simulink model "four_quad_formation_270714"  (R2012b)
settings: Solver=ode5  StartTime=0.0  StopTime=inf  FixedStep=sample_time  RelTol=1e-3
InitFcn:
  | sample_time=0.005;%0.004;%0.0025;%0.02;
  | sample_time_Vicon = 0.005;
  | DeltaT = 0.02;
  | g = 9.81;
  | H0 = g%0.3165;
  | Kl = 1;
  | 
  | Q6_mass = 0.8;
  | 
  | Q6_Omega_r = 1.2; %for horizon ref
  | Q6_Zeta_r = 0.707; %for horizon ref
  | Q6_Omega_r_h = 2;%for vertical ref
  | Q6_Zeta_r_h = 0.7; %for vertical ref
  | 
  | 
  | Q6_Omega = 1.5; %for horizon control
  | Q6_Zeta = 0.507; %for horizon control
  | Q6_Omega_h= 2 %for vertical control
  | Q6_Zeta_h = 0.5; %for vertical control
  | 
  | 
  | Q6_acc_max = 5;%horizontal max acc
  | Q6_acc_max_h = 5;%horizontal max acc
  | 
  | omega_circle = 10*pi/180;
  | 
  | omega_h = 0.1;%Ascending speed
  | PI = pi;
  | Circle_R = 2;
  | 
  | 
  | MAX_Height = -2;
  | 
  | 
  | % for NN
  | n = 5;
  | r = 3;
  | n2 = 5;
  | NN_ST = 0.02;
  | 
  | GAMA_V = 6;
  | gama_V_e = 0.01;
  | 
  | GAMA_W = GAMA_V;
  | gama_W_e =0.01;
  | 
  | % deadzone
  | NN_Deadzone_Z = 0;
  | 
  | % inputs nomalizaton parameters
  | NN_Z_y_min = -3;
  | NN_Z_y_max = 0.5;
  | 
  | NN_Z_v_max = 8;
  | NN_Z_v_min = -NN_Z_v_max;
  | 
  | % alpha = 0.034;
  | alpha = 1;
  | % c_f = 0.0015;
  | c_f = 0.001;
  | c_y_tilt = 1*0.5;
libraries: X330_Control x20, simulink x8
settings Model: Creator=ttcl3  LastModifiedBy=Vicon
settings SolverCC: MaxConsecutiveMinStep=auto
settings DataIOCC: SignalLoggingSaveFormat=ModelDataLogs
settings DebuggingCC: MultiTaskRateTransMsg=warning  FcnCallInpInsideContextMsg=UseLocalSettings
settings SFSimCC: SimParseCustomCode=off
settings GRTTargetCC: CombineOutputUpdateFcns=off  GRTInterface=on

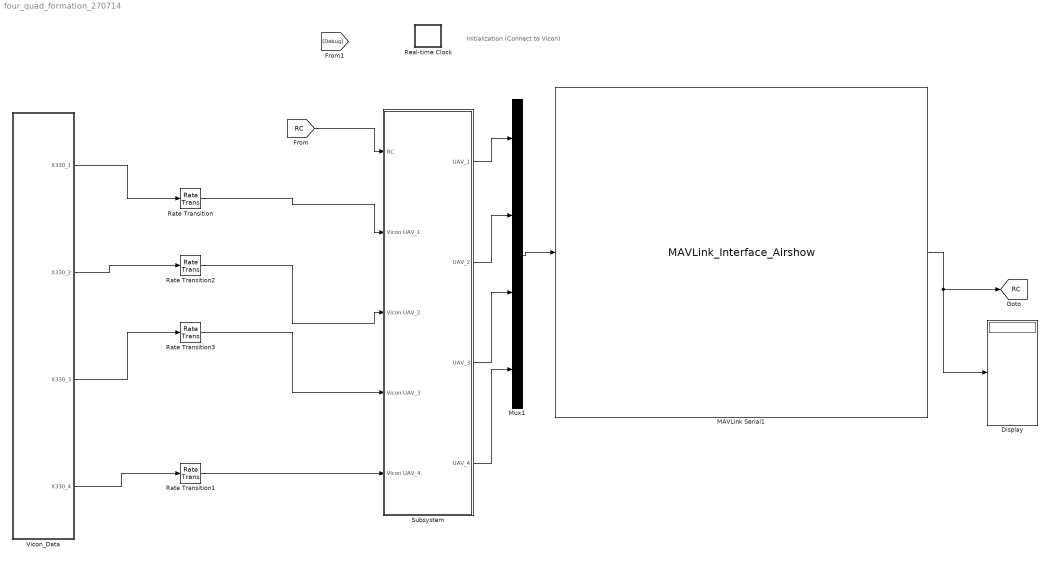
== system four_quad_formation_270714 ==
  note: Initialization
      | (Connect to Vicon)
  Display : Display
  MAVLink Serial1 : S-Function  FunctionName=MAVLink_Interface_Airshow  Parameters=COM_Port,Baud_Rate,MSG_INPUT,MSG_OUTPUT  EnableBusSupport=off  mask{COM_Port='COM6', Baud_Rate=57600, ATTITUDE_OUT=off, RC_SCALED=on, Quads_1=off, Quads_2=off, Quads_3=off, Quads_4=on, Quads_5=off, Quads_6=off}
      mask prompts: COM_Port "COM Port"; Baud_Rate "Baud Rate"; ATTITUDE_OUT "DEBUG"; RC_SCALED "RC CHANNELS SCALED"; Quads_1 "1 Quad"; Quads_2 "2 Quad"; Quads_3 "3 Quad"; Quads_4 "4 Quad"; Quads_5 "5 Quad"; Quads_6 "6 Quad"
      mask init:
      | MSG_ID_NUM_INPUT = [ uint8(221) uint8(222) uint8(223) uint8(224) uint8(225) uint8(226)];
      | MSG_ID_NAME_INPUT = [Quads_1 Quads_2 Quads_3 Quads_4 Quads_5 Quads_6];
      | 
      | MSG_ID_NUM_OUTPUT = [uint8(34) uint8(30)];
      | MSG_ID_NAME_OUTPUT = [RC_SCALED ATTITUDE_OUT ];
      | 
      | idx_input = find(MSG_ID_NAME_INPUT);
      | MSG_INPUT = MSG_ID_NUM_INPUT(idx_input);
      | 
      | idx_output = find(MSG_ID_NAME_OUTPUT);
      | MSG_OUTPUT = MSG_ID_NUM_OUTPUT(idx_output);
      mask Display:
      | % Block image
      | image(imread('10-inch Quad Heat Map.png'));
      | 
      | %Label block
      | fprintf('MAVLink Serial\n%s\n%dbps', COM_Port,  Baud_Rate)
      | 
      | 
      | %Label input ports
      | 
      | in = 1;
      | if (Quads_1 == 1)
      |     port_label('input', in, 'Quads_1');
      |     in = in + 1;
      | end
      | 
      | if (Quads_2 == 1)
      |     port_label('input', in, 'Quads_2');
      |     in = in + 1;
      | end
      | 
      | if (Quads_3 == 1)
      |     port_label('input', in, 'Quads_3');
      |     in = in + 1;
      | end
      | 
      | if (Quads_4 == 1)
      |     port_label('input', in, 'Quads_4');
      |     in = in + 1;
      | end
      | 
      | if (Quads_5 == 1)
      |     port_label('input', in, 'Quads_5');
      |     in = in + 1;
      | end
      | 
      | 
      | if (Quads_6 == 1)
      |     port_label('input', in, 'Quads_6');
      |     in = in + 1;
      | end
      | %Label output ports
      | 
      | out = 1;
      | if (RC_SCALED == 1)
      |     port_label('output', out, 'RC CMD');
      |     out = out + 1;
      | end
      | 
      | if (ATTITUDE_OUT == 1)
      |     port_label('output', out, 'DEBUG');
      |     out = out + 1;
      | end
  Mux1 : Mux
  Rate Transition{,1..3} (4 alike) : RateTransition  OutPortSampleTime=0.02
  Real-time Clock : Subsystem  mask(Real-time Clock){sample_time=0.02, tolerance=1}
      mask prompts: sample_time "Synchronize with real-time every n seconds:"; tolerance "Real-time warning tolerance (seconds):"
      mask help: Real-time Synchronization Block
      mask Help: This block synchronizes simulation time with the PC real-time clock or UNIX system clock. The first dialog entry is the period at which the clock is checked to insure real-time synchronization. The second dialog entry is the number of seconds that the simulation time must be within real-time before a warning is printed.
      mask Display: plot(0,0,100,100,[40,60,60,54,54,64,69,76,82,77,81,83,83,81,78,74,70,64,57,49,41,35,32,30,30,31,34,40,47,47,40,40],[90,90,85,85,80,79,76,87,80,70,64,57,49,41,33,28,24,22,21,23,25,31,37,46,56,65,73,78,80,85,85,90],[69,53,53],[64,50,73])
  Subsystem : Subsystem
  Vicon_Data : Subsystem
  tag scope: RC=global
  wires:
  MAVLink Serial1/1 -> [RC], Display/1
  Mux1/1 -> MAVLink Serial1/1
  Vicon_Data/1(X330_1) -> Rate Transition/1
  Vicon_Data/2(X330_2) -> Rate Transition2/1
  Vicon_Data/3(X330_3) -> Rate Transition3/1
  Rate Transition/1 -> Subsystem/2(Vicon UAV_1)
  [RC] -> Subsystem/1(RC)
  Rate Transition2/1 -> Subsystem/3(Vicon UAV_2)
  Rate Transition3/1 -> Subsystem/4(Vicon UAV_3)
  Subsystem/1(UAV_1) -> Mux1/1
  Subsystem/2(UAV_2) -> Mux1/2
  Subsystem/3(UAV_3) -> Mux1/3
  Rate Transition1/1 -> Subsystem/5(Vicon UAV_4)
  Vicon_Data/4(X330_4) -> Rate Transition1/1
  Subsystem/4(UAV_4) -> Mux1/4

== system four_quad_formation_270714/Real-time Clock ==
  Real-time Clock : S-Function  FunctionName=rtclock  Parameters=sample_time, tolerance  EnableBusSupport=off

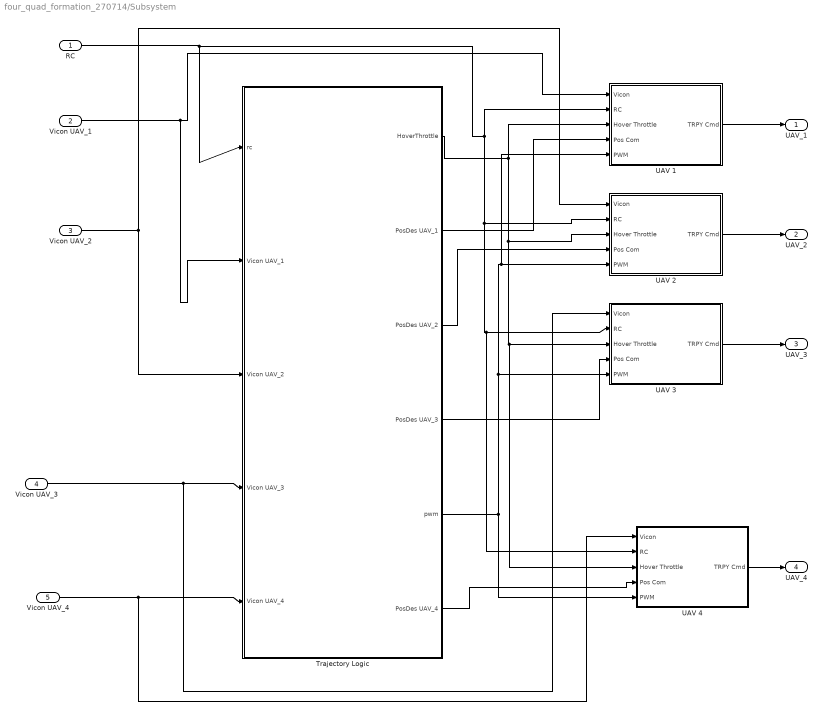
== system four_quad_formation_270714/Subsystem ==
  RC : Inport
  Vicon UAV_1 : Inport  Port=2
  Vicon UAV_2 : Inport  Port=3
  Vicon UAV_3 : Inport  Port=4
  Vicon UAV_4 : Inport  Port=5
  Trajectory Logic : Subsystem
  UAV 1 : Subsystem
  UAV 2 : Subsystem
  UAV 3 : Subsystem
  UAV 4 : Subsystem
  UAV_1 : Outport
  UAV_2 : Outport  Port=2
  UAV_3 : Outport  Port=3
  UAV_4 : Outport  Port=4
  wires:
  RC/1 -> Trajectory Logic/1(rc), UAV 1/2(RC), UAV 4/2(RC), UAV 3/2(RC), UAV 2/2(RC)
  Vicon UAV_1/1 -> UAV 1/1(Vicon), Trajectory Logic/2(Vicon UAV_1)
  UAV 1/1(TRPY Cmd) -> UAV_1/1
  Trajectory Logic/1(HoverThrottle) -> UAV 1/3(Hover Throttle), UAV 4/3(Hover Throttle), UAV 3/3(Hover Throttle), UAV 2/3(Hover Throttle)
  Trajectory Logic/2(PosDes UAV_1) -> UAV 1/4(Pos Com)
  Vicon UAV_2/1 -> Trajectory Logic/3(Vicon UAV_2), UAV 2/1(Vicon)
  Vicon UAV_3/1 -> UAV 3/1(Vicon), Trajectory Logic/4(Vicon UAV_3)
  Trajectory Logic/3(PosDes UAV_2) -> UAV 2/4(Pos Com)
  Trajectory Logic/4(PosDes UAV_3) -> UAV 3/4(Pos Com)
  UAV 2/1(TRPY Cmd) -> UAV_2/1
  UAV 3/1(TRPY Cmd) -> UAV_3/1
  Trajectory Logic/5(pwm) -> UAV 4/5(PWM), UAV 1/5(PWM), UAV 2/5(PWM), UAV 3/5(PWM)
  UAV 4/1(TRPY Cmd) -> UAV_4/1
  Vicon UAV_4/1 -> UAV 4/1(Vicon), Trajectory Logic/5(Vicon UAV_4)
  Trajectory Logic/6(PosDes UAV_4) -> UAV 4/4(Pos Com)

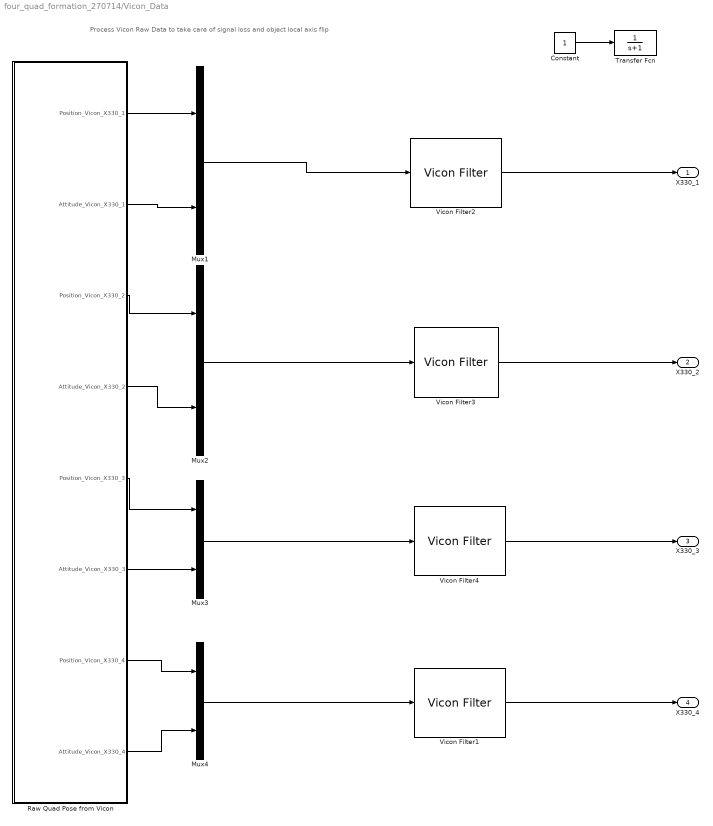
== system four_quad_formation_270714/Vicon_Data ==
  note: Process Vicon Raw Data to take care of signal loss and object local axis flip
  Constant : Constant  SampleTime=5
  Mux{1..4} (4 alike) : Mux  Inputs=2
  Raw Quad Pose from Vicon : Subsystem
  Transfer Fcn : TransferFcn  Denominator=[1 1]
  Vicon Filter{1..4} (4 alike) : X330_Control/Vicon Filter
  X330_1 : Outport
  X330_2 : Outport  Port=2
  X330_3 : Outport  Port=3
  X330_4 : Outport  Port=4
  wires:
  Vicon Filter2/1 -> X330_1/1
  Vicon Filter3/1 -> X330_2/1
  Vicon Filter4/1 -> X330_3/1
  Constant/1 -> Transfer Fcn/1
  Raw Quad Pose from Vicon/1(Position_Vicon_X330_1) -> Mux1/1
  Raw Quad Pose from Vicon/2(Attitude_Vicon_X330_1) -> Mux1/2
  Raw Quad Pose from Vicon/3(Position_Vicon_X330_2) -> Mux2/1
  Raw Quad Pose from Vicon/4(Attitude_Vicon_X330_2) -> Mux2/2
  Raw Quad Pose from Vicon/5(Position_Vicon_X330_3) -> Mux3/1
  Raw Quad Pose from Vicon/6(Attitude_Vicon_X330_3) -> Mux3/2
  Mux1/1 -> Vicon Filter2/1
  Mux2/1 -> Vicon Filter3/1
  Mux3/1 -> Vicon Filter4/1
  Vicon Filter1/1 -> X330_4/1
  Mux4/1 -> Vicon Filter1/1
  Raw Quad Pose from Vicon/7(Position_Vicon_X330_4) -> Mux4/1
  Raw Quad Pose from Vicon/8(Attitude_Vicon_X330_4) -> Mux4/2

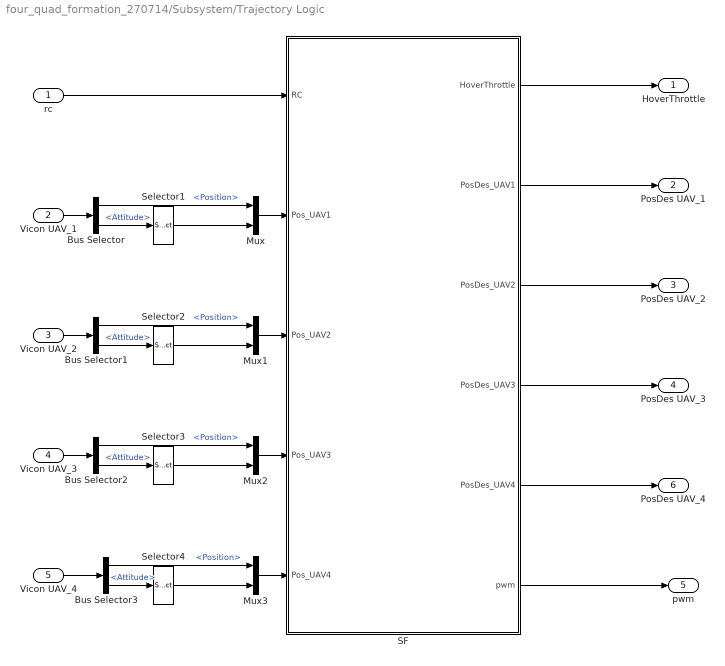
== system four_quad_formation_270714/Subsystem/Trajectory Logic ==
  rc : Inport
  Vicon UAV_1 : Inport  Port=2
  Vicon UAV_2 : Inport  Port=3
  Vicon UAV_3 : Inport  Port=4
  Vicon UAV_4 : Inport  Port=5
  " SF" : Stateflow chart  TreatAsAtomicUnit=on
  Bus Selector{,1..3} (4 alike) : BusSelector  OutputSignals=Position,Attitude
  Mux{,1..3} (4 alike) : Mux  Inputs=2
  Selector{1..4} (4 alike) : Selector  InputPortWidth=3  IndexOptions=Index vector (dialog)  Indices=[3]  OutputSizes=1
  HoverThrottle : Outport
  PosDes UAV_1 : Outport  Port=2
  PosDes UAV_2 : Outport  Port=3
  PosDes UAV_3 : Outport  Port=4
  pwm : Outport  Port=5
  PosDes UAV_4 : Outport  Port=6
  wires:
  Mux/1 -> " SF"/2(Pos_UAV1)
  Selector1/1 -> Mux/2
  Bus Selector/2 -> Selector1/1  "<Attitude>"
  Bus Selector/1 -> Mux/1  "<Position>"
  " SF"/1(HoverThrottle) -> HoverThrottle/1
  rc/1 -> " SF"/1(RC)
  " SF"/2(PosDes_UAV1) -> PosDes UAV_1/1
  Vicon UAV_1/1 -> Bus Selector/1
  Mux1/1 -> " SF"/3(Pos_UAV2)
  Selector2/1 -> Mux1/2
  Bus Selector1/2 -> Selector2/1  "<Attitude>"
  Bus Selector1/1 -> Mux1/1  "<Position>"
  Vicon UAV_2/1 -> Bus Selector1/1
  Selector3/1 -> Mux2/2
  Bus Selector2/2 -> Selector3/1  "<Attitude>"
  Bus Selector2/1 -> Mux2/1  "<Position>"
  Vicon UAV_3/1 -> Bus Selector2/1
  Mux2/1 -> " SF"/4(Pos_UAV3)
  " SF"/3(PosDes_UAV2) -> PosDes UAV_2/1
  " SF"/4(PosDes_UAV3) -> PosDes UAV_3/1
  " SF"/6(pwm) -> pwm/1
  Selector4/1 -> Mux3/2
  Bus Selector3/2 -> Selector4/1  "<Attitude>"
  Bus Selector3/1 -> Mux3/1  "<Position>"
  Vicon UAV_4/1 -> Bus Selector3/1
  Mux3/1 -> " SF"/5(Pos_UAV4)
  " SF"/5(PosDes_UAV4) -> PosDes UAV_4/1

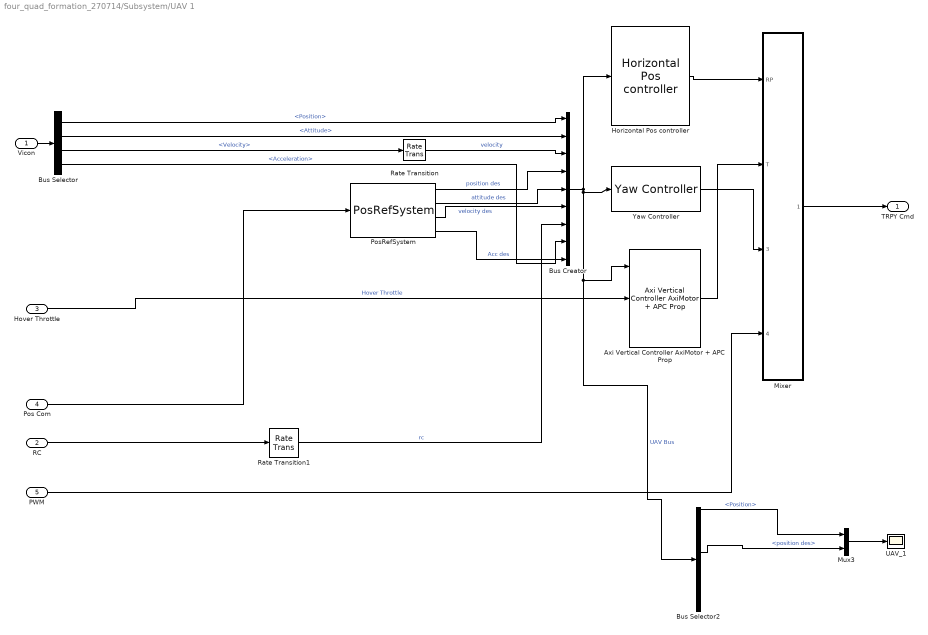
== system four_quad_formation_270714/Subsystem/UAV 1 ==
  Vicon : Inport
  RC : Inport  Port=2
  Hover Throttle : Inport  Port=3
  Pos Com : Inport  Port=4
  PWM : Inport  Port=5
  Axi Vertical Controller AxiMotor + APC Prop : X330_Control/Axi Vertical Controller AxiMotor + APC Prop  Omega_h=Q6_Omega_h  Zeta_h=Q6_Zeta_h  PID_I_h=1  mass=Q6_mass
  Bus Creator : BusCreator  Inputs=9
  Bus Selector : BusSelector  OutputSignals=Position,Attitude,Velocity,Acceleration
  Bus Selector2 : BusSelector  OutputSignals=Position,Attitude,velocity,position des,attitude des,velocity des,rc,Acc des
  Horizontal Pos controller : X330_Control/Horizontal Pos controller  Max_RP=60  Omega=Q6_Omega  PID_i=0.5  Zeta=Q6_Zeta
  Mixer : Subsystem
  Mux3 : Mux  Inputs=2
  PosRefSystem : X330_Control/PosRefSystem  Omega_r=Q6_Omega_r  Zeta_r=Q6_Zeta_r  Acc_Max=Q6_acc_max  Omega_h_r=Q6_Omega_r_h  Zeta_h_r=Q6_Zeta_r_h  Acc_h_Max=Q6_acc_max_h
      link override Saturation: LowerLimit=-3.0
  Rate Transition : RateTransition  OutPortSampleTime=0.02
  Rate Transition1 : RateTransition  OutPortSampleTime=0.02
  UAV_1 : Scope
      settings: TimeRange=10  YMin=-2.5  YMax=2
  Yaw Controller : X330_Control/Yaw Controller
  TRPY Cmd : Outport
  wires:
  Mux3/1 -> UAV_1/1
  Bus Selector2/4 -> Mux3/2  "<position des>"
  Bus Selector2/1 -> Mux3/1  "<Position>"
  RC/1 -> Rate Transition1/1
  PosRefSystem/4 -> Bus Creator/9  "Acc des"
  Vicon/1 -> Bus Selector/1
  Bus Selector/3 -> Rate Transition/1  "<Velocity>"
  Bus Selector/2 -> Bus Creator/2  "<Attitude>"
  Bus Selector/1 -> Bus Creator/1  "<Position>"
  Hover Throttle/1 -> Axi Vertical Controller AxiMotor + APC Prop/2  "Hover Throttle"
  PosRefSystem/3 -> Bus Creator/6  "velocity des"
  PosRefSystem/2 -> Bus Creator/5  "attitude des"
  PosRefSystem/1 -> Bus Creator/4  "position des"
  Bus Selector/4 -> Bus Creator/8  "<Acceleration>"
  Axi Vertical Controller AxiMotor + APC Prop/1 -> Mixer/2(T)
  Yaw Controller/1 -> Mixer/3(Yaw rate)
  Bus Creator/1 -> Yaw Controller/1, Bus Selector2/1, Axi Vertical Controller AxiMotor + APC Prop/1, Horizontal Pos controller/1  "UAV Bus"
  Rate Transition1/1 -> Bus Creator/7  "rc"
  Rate Transition/1 -> Bus Creator/3  "velocity"
  Horizontal Pos controller/1 -> Mixer/1(RP)
  Mixer/1(UAV_1) -> TRPY Cmd/1
  Pos Com/1 -> PosRefSystem/1
  PWM/1 -> Mixer/4(PWM)

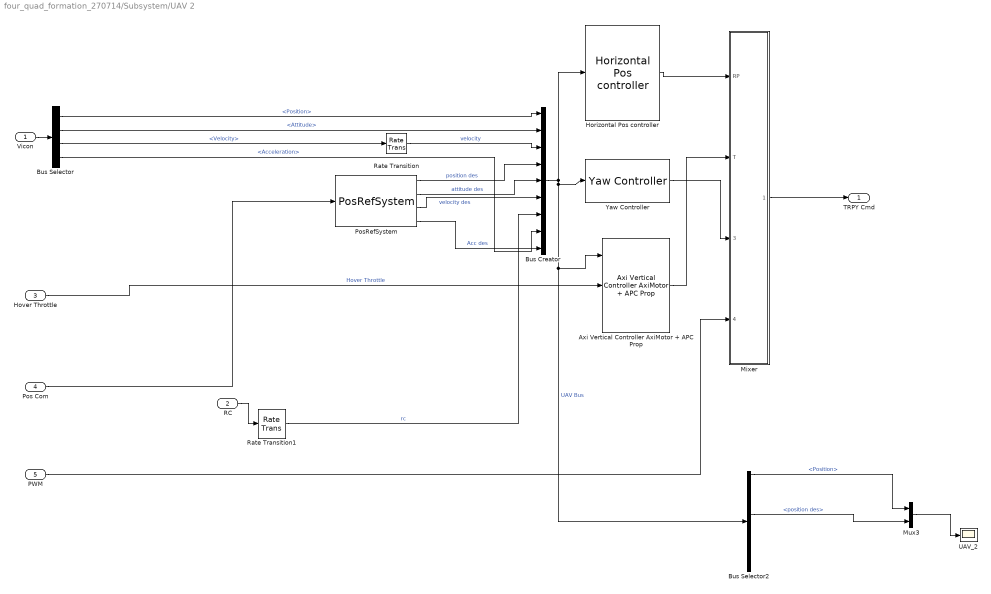
== system four_quad_formation_270714/Subsystem/UAV 2 ==
  Vicon : Inport
  RC : Inport  Port=2
  Hover Throttle : Inport  Port=3
  Pos Com : Inport  Port=4
  PWM : Inport  Port=5
  Axi Vertical Controller AxiMotor + APC Prop : X330_Control/Axi Vertical Controller AxiMotor + APC Prop  Omega_h=Q6_Omega_h  Zeta_h=Q6_Zeta_h  PID_I_h=1  mass=Q6_mass
  Bus Creator : BusCreator  Inputs=9
  Bus Selector : BusSelector  OutputSignals=Position,Attitude,Velocity,Acceleration
  Bus Selector2 : BusSelector  OutputSignals=Position,Attitude,velocity,position des,attitude des,velocity des,rc,Acc des
  Horizontal Pos controller : X330_Control/Horizontal Pos controller  Max_RP=60  Omega=Q6_Omega  PID_i=0.5  Zeta=Q6_Zeta
  Mixer : Subsystem
  Mux3 : Mux  Inputs=2
  PosRefSystem : X330_Control/PosRefSystem  Omega_r=Q6_Omega_r  Zeta_r=Q6_Zeta_r  Acc_Max=Q6_acc_max  Omega_h_r=Q6_Omega_r_h  Zeta_h_r=Q6_Zeta_r_h  Acc_h_Max=Q6_acc_max_h
      link override Saturation: LowerLimit=-3.0
  Rate Transition : RateTransition  OutPortSampleTime=0.02
  Rate Transition1 : RateTransition  OutPortSampleTime=0.02
  UAV_2 : Scope
      settings: TimeRange=10  YMin=-0.55  YMax=0.1  SaveName=ScopeData2
  Yaw Controller : X330_Control/Yaw Controller
  TRPY Cmd : Outport
  wires:
  Pos Com/1 -> PosRefSystem/1
  Mixer/1(UAV_1) -> TRPY Cmd/1
  Horizontal Pos controller/1 -> Mixer/1(RP)
  Rate Transition/1 -> Bus Creator/3  "velocity"
  Rate Transition1/1 -> Bus Creator/7  "rc"
  Yaw Controller/1 -> Mixer/3(Yaw rate)
  Axi Vertical Controller AxiMotor + APC Prop/1 -> Mixer/2(T)
  Bus Selector/4 -> Bus Creator/8  "<Acceleration>"
  PosRefSystem/1 -> Bus Creator/4  "position des"
  PosRefSystem/2 -> Bus Creator/5  "attitude des"
  PosRefSystem/3 -> Bus Creator/6  "velocity des"
  Hover Throttle/1 -> Axi Vertical Controller AxiMotor + APC Prop/2  "Hover Throttle"
  Bus Selector/1 -> Bus Creator/1  "<Position>"
  Bus Selector/2 -> Bus Creator/2  "<Attitude>"
  Bus Selector/3 -> Rate Transition/1  "<Velocity>"
  Vicon/1 -> Bus Selector/1
  PosRefSystem/4 -> Bus Creator/9  "Acc des"
  RC/1 -> Rate Transition1/1
  PWM/1 -> Mixer/4(PWM)
  Mux3/1 -> UAV_2/1
  Bus Selector2/4 -> Mux3/2  "<position des>"
  Bus Selector2/1 -> Mux3/1  "<Position>"
  Bus Creator/1 -> Horizontal Pos controller/1, Bus Selector2/1, Axi Vertical Controller AxiMotor + APC Prop/1, Yaw Controller/1  "UAV Bus"

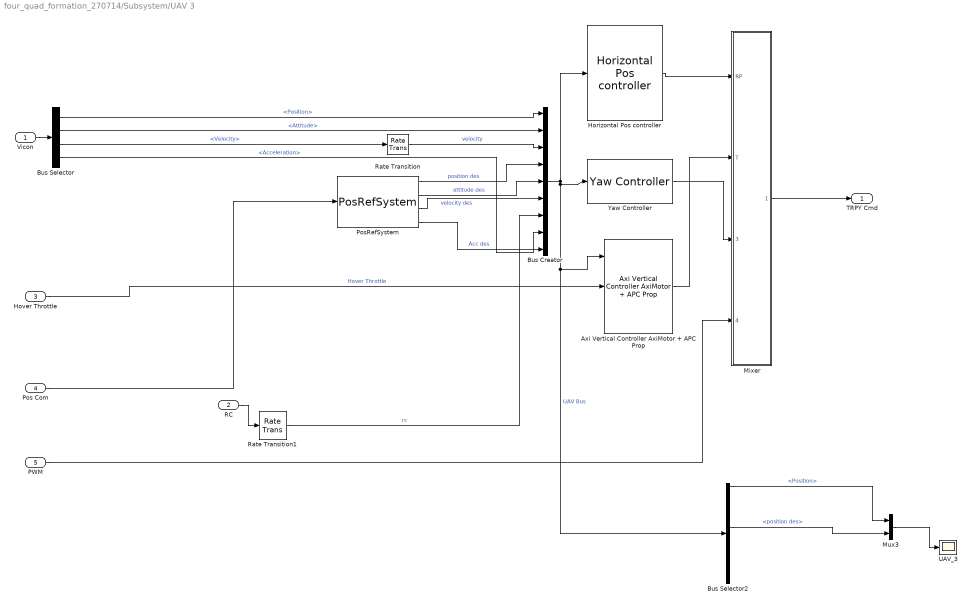
== system four_quad_formation_270714/Subsystem/UAV 3 ==
  Vicon : Inport
  RC : Inport  Port=2
  Hover Throttle : Inport  Port=3
  Pos Com : Inport  Port=4
  PWM : Inport  Port=5
  Axi Vertical Controller AxiMotor + APC Prop : X330_Control/Axi Vertical Controller AxiMotor + APC Prop  Omega_h=Q6_Omega_h  Zeta_h=Q6_Zeta_h  PID_I_h=1  mass=Q6_mass
  Bus Creator : BusCreator  Inputs=9
  Bus Selector : BusSelector  OutputSignals=Position,Attitude,Velocity,Acceleration
  Bus Selector2 : BusSelector  OutputSignals=Position,Attitude,velocity,position des,attitude des,velocity des,rc,Acc des
  Horizontal Pos controller : X330_Control/Horizontal Pos controller  Max_RP=60  Omega=Q6_Omega  PID_i=0.5  Zeta=Q6_Zeta
  Mixer : Subsystem
  Mux3 : Mux  Inputs=2
  PosRefSystem : X330_Control/PosRefSystem  Omega_r=Q6_Omega_r  Zeta_r=Q6_Zeta_r  Acc_Max=Q6_acc_max  Omega_h_r=Q6_Omega_r_h  Zeta_h_r=Q6_Zeta_r_h  Acc_h_Max=Q6_acc_max_h
      link override Saturation: LowerLimit=-3.0
  Rate Transition : RateTransition  OutPortSampleTime=0.02
  Rate Transition1 : RateTransition  OutPortSampleTime=0.02
  UAV_3 : Scope
      settings: TimeRange=10  YMin=-1.7  YMax=0
  Yaw Controller : X330_Control/Yaw Controller
  TRPY Cmd : Outport
  wires:
  RC/1 -> Rate Transition1/1
  PosRefSystem/4 -> Bus Creator/9  "Acc des"
  Vicon/1 -> Bus Selector/1
  Bus Selector/3 -> Rate Transition/1  "<Velocity>"
  Bus Selector/2 -> Bus Creator/2  "<Attitude>"
  Bus Selector/1 -> Bus Creator/1  "<Position>"
  Hover Throttle/1 -> Axi Vertical Controller AxiMotor + APC Prop/2  "Hover Throttle"
  PosRefSystem/3 -> Bus Creator/6  "velocity des"
  PosRefSystem/2 -> Bus Creator/5  "attitude des"
  PosRefSystem/1 -> Bus Creator/4  "position des"
  Bus Selector/4 -> Bus Creator/8  "<Acceleration>"
  Axi Vertical Controller AxiMotor + APC Prop/1 -> Mixer/2(T)
  Yaw Controller/1 -> Mixer/3(Yaw rate)
  Rate Transition1/1 -> Bus Creator/7  "rc"
  Rate Transition/1 -> Bus Creator/3  "velocity"
  Horizontal Pos controller/1 -> Mixer/1(RP)
  Mixer/1(UAV_1) -> TRPY Cmd/1
  Pos Com/1 -> PosRefSystem/1
  PWM/1 -> Mixer/4(PWM)
  Mux3/1 -> UAV_3/1
  Bus Selector2/4 -> Mux3/2  "<position des>"
  Bus Selector2/1 -> Mux3/1  "<Position>"
  Bus Creator/1 -> Yaw Controller/1, Bus Selector2/1, Axi Vertical Controller AxiMotor + APC Prop/1, Horizontal Pos controller/1  "UAV Bus"

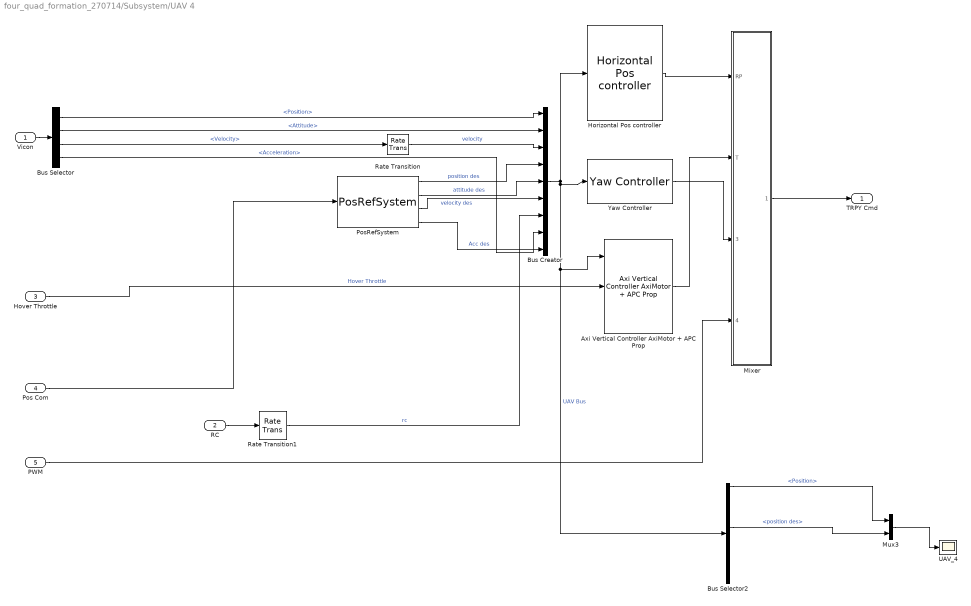
== system four_quad_formation_270714/Subsystem/UAV 4 ==
  Vicon : Inport
  RC : Inport  Port=2
  Hover Throttle : Inport  Port=3
  Pos Com : Inport  Port=4
  PWM : Inport  Port=5
  Axi Vertical Controller AxiMotor + APC Prop : X330_Control/Axi Vertical Controller AxiMotor + APC Prop  Omega_h=Q6_Omega_h  Zeta_h=Q6_Zeta_h  PID_I_h=1  mass=Q6_mass
  Bus Creator : BusCreator  Inputs=9
  Bus Selector : BusSelector  OutputSignals=Position,Attitude,Velocity,Acceleration
  Bus Selector2 : BusSelector  OutputSignals=Position,Attitude,velocity,position des,attitude des,velocity des,rc,Acc des
  Horizontal Pos controller : X330_Control/Horizontal Pos controller  Max_RP=60  Omega=Q6_Omega  PID_i=0.5  Zeta=Q6_Zeta
  Mixer : Subsystem
  Mux3 : Mux  Inputs=2
  PosRefSystem : X330_Control/PosRefSystem  Omega_r=Q6_Omega_r  Zeta_r=Q6_Zeta_r  Acc_Max=Q6_acc_max  Omega_h_r=Q6_Omega_r_h  Zeta_h_r=Q6_Zeta_r_h  Acc_h_Max=Q6_acc_max_h
      link override Saturation: LowerLimit=-3.0
  Rate Transition : RateTransition  OutPortSampleTime=0.02
  Rate Transition1 : RateTransition  OutPortSampleTime=0.02
  UAV_4 : Scope
      settings: TimeRange=10  YMin=-2.75  YMax=2.25
  Yaw Controller : X330_Control/Yaw Controller
  TRPY Cmd : Outport
  wires:
  Bus Creator/1 -> Horizontal Pos controller/1, Axi Vertical Controller AxiMotor + APC Prop/1, Bus Selector2/1, Yaw Controller/1  "UAV Bus"
  Bus Selector2/1 -> Mux3/1  "<Position>"
  Bus Selector2/4 -> Mux3/2  "<position des>"
  Mux3/1 -> UAV_4/1
  PWM/1 -> Mixer/4(PWM)
  Pos Com/1 -> PosRefSystem/1
  Mixer/1(UAV_1) -> TRPY Cmd/1
  Horizontal Pos controller/1 -> Mixer/1(RP)
  Rate Transition/1 -> Bus Creator/3  "velocity"
  Rate Transition1/1 -> Bus Creator/7  "rc"
  Yaw Controller/1 -> Mixer/3(Yaw rate)
  Axi Vertical Controller AxiMotor + APC Prop/1 -> Mixer/2(T)
  Bus Selector/4 -> Bus Creator/8  "<Acceleration>"
  PosRefSystem/1 -> Bus Creator/4  "position des"
  PosRefSystem/2 -> Bus Creator/5  "attitude des"
  PosRefSystem/3 -> Bus Creator/6  "velocity des"
  Hover Throttle/1 -> Axi Vertical Controller AxiMotor + APC Prop/2  "Hover Throttle"
  Bus Selector/1 -> Bus Creator/1  "<Position>"
  Bus Selector/2 -> Bus Creator/2  "<Attitude>"
  Bus Selector/3 -> Rate Transition/1  "<Velocity>"
  Vicon/1 -> Bus Selector/1
  PosRefSystem/4 -> Bus Creator/9  "Acc des"
  RC/1 -> Rate Transition1/1

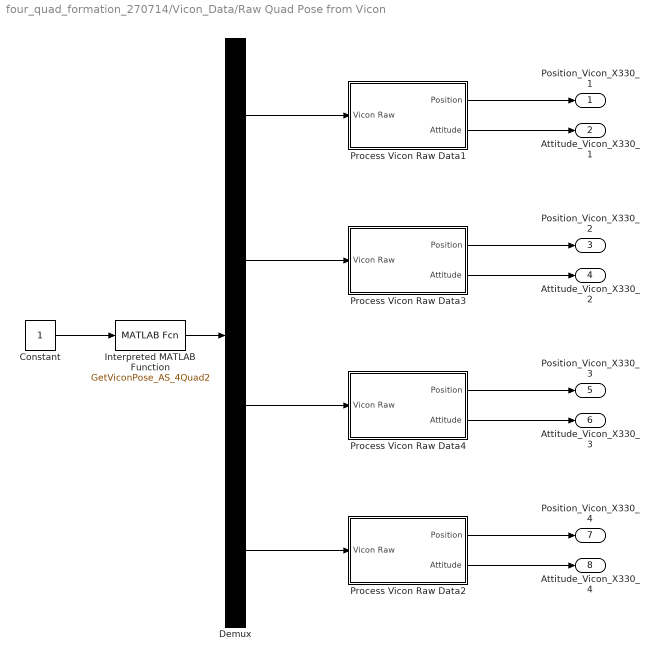
== system four_quad_formation_270714/Vicon_Data/Raw Quad Pose from Vicon ==
  Constant : Constant  SampleTime=sample_time
  Demux : Demux
  Interpreted MATLAB Function : MATLABFcn  MATLABFcn=GetViconPose_AS_4Quad2
  Process Vicon Raw Data1 : Subsystem
  Process Vicon Raw Data2 : Subsystem
  Process Vicon Raw Data3 : Subsystem
  Process Vicon Raw Data4 : Subsystem
  Position_Vicon_X330_1 : Outport
  Attitude_Vicon_X330_1 : Outport  Port=2
  Position_Vicon_X330_2 : Outport  Port=3
  Attitude_Vicon_X330_2 : Outport  Port=4
  Position_Vicon_X330_3 : Outport  Port=5
  Attitude_Vicon_X330_3 : Outport  Port=6
  Position_Vicon_X330_4 : Outport  Port=7
  Attitude_Vicon_X330_4 : Outport  Port=8
  wires:
  Interpreted MATLAB Function/1 -> Demux/1
  Constant/1 -> Interpreted MATLAB Function/1
  Process Vicon Raw Data1/2(Attitude) -> Attitude_Vicon_X330_1/1
  Process Vicon Raw Data1/1(Position) -> Position_Vicon_X330_1/1
  Process Vicon Raw Data3/2(Attitude) -> Attitude_Vicon_X330_2/1
  Process Vicon Raw Data3/1(Position) -> Position_Vicon_X330_2/1
  Process Vicon Raw Data4/2(Attitude) -> Attitude_Vicon_X330_3/1
  Process Vicon Raw Data4/1(Position) -> Position_Vicon_X330_3/1
  Demux/1 -> Process Vicon Raw Data1/1(Vicon Raw)
  Demux/2 -> Process Vicon Raw Data3/1(Vicon Raw)
  Demux/3 -> Process Vicon Raw Data4/1(Vicon Raw)
  Process Vicon Raw Data2/2(Attitude) -> Attitude_Vicon_X330_4/1
  Process Vicon Raw Data2/1(Position) -> Position_Vicon_X330_4/1
  Demux/4 -> Process Vicon Raw Data2/1(Vicon Raw)

== system four_quad_formation_270714/Subsystem/UAV 1/Mixer ==
  RP : Inport
  T : Inport  Port=2
  Yaw rate : Inport  Port=3
  PWM : Inport  Port=4
  Gain : Gain  Gain=180/pi
  Mode : Constant  SampleTime=0.02
  Mux1 : Mux  Inputs=5
  "[-1, 1]" : Fcn  Expr=u(1)*2-1
  UAV_1 : Outport
  wires:
  "[-1, 1]"/1 -> Mux1/1
  Gain/1 -> Mux1/2
  Mode/1 -> Mux1/4
  Yaw rate/1 -> Mux1/3
  RP/1 -> Gain/1
  T/1 -> "[-1, 1]"/1
  Mux1/1 -> UAV_1/1
  PWM/1 -> Mux1/5

== system four_quad_formation_270714/Subsystem/UAV 2/Mixer ==
  RP : Inport
  T : Inport  Port=2
  Yaw rate : Inport  Port=3
  PWM : Inport  Port=4
  Gain : Gain  Gain=180/pi
  Mode : Constant  SampleTime=0.02
  Mux1 : Mux  Inputs=5
  "[-1, 1]" : Fcn  Expr=u(1)*2-1
  UAV_1 : Outport
  wires:
  PWM/1 -> Mux1/5
  Mux1/1 -> UAV_1/1
  T/1 -> "[-1, 1]"/1
  RP/1 -> Gain/1
  Yaw rate/1 -> Mux1/3
  Mode/1 -> Mux1/4
  Gain/1 -> Mux1/2
  "[-1, 1]"/1 -> Mux1/1

== system four_quad_formation_270714/Subsystem/UAV 3/Mixer ==
  RP : Inport
  T : Inport  Port=2
  Yaw rate : Inport  Port=3
  PWM : Inport  Port=4
  Gain : Gain  Gain=180/pi
  Mode : Constant  SampleTime=0.02
  Mux1 : Mux  Inputs=5
  "[-1, 1]" : Fcn  Expr=u(1)*2-1
  UAV_1 : Outport
  wires:
  "[-1, 1]"/1 -> Mux1/1
  Gain/1 -> Mux1/2
  Mode/1 -> Mux1/4
  Yaw rate/1 -> Mux1/3
  RP/1 -> Gain/1
  T/1 -> "[-1, 1]"/1
  Mux1/1 -> UAV_1/1
  PWM/1 -> Mux1/5

== system four_quad_formation_270714/Subsystem/UAV 4/Mixer ==
  RP : Inport
  T : Inport  Port=2
  Yaw rate : Inport  Port=3
  PWM : Inport  Port=4
  Gain : Gain  Gain=180/pi
  Mode : Constant  SampleTime=0.02
  Mux1 : Mux  Inputs=5
  "[-1, 1]" : Fcn  Expr=u(1)*2-1
  UAV_1 : Outport
  wires:
  PWM/1 -> Mux1/5
  Mux1/1 -> UAV_1/1
  T/1 -> "[-1, 1]"/1
  RP/1 -> Gain/1
  Yaw rate/1 -> Mux1/3
  Mode/1 -> Mux1/4
  Gain/1 -> Mux1/2
  "[-1, 1]"/1 -> Mux1/1

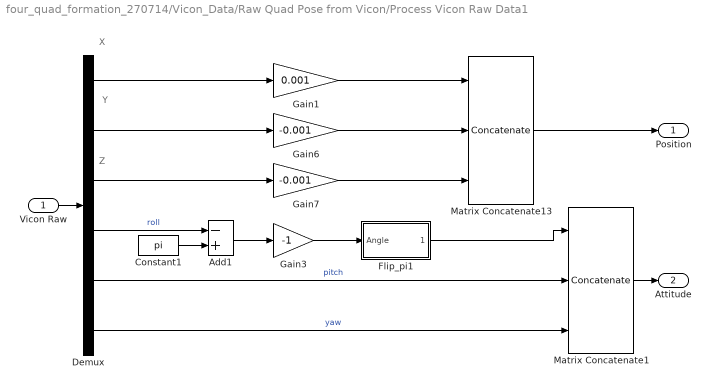
== system four_quad_formation_270714/Vicon_Data/Raw Quad Pose from Vicon/Process Vicon Raw Data1 ==
  note: X
  note: Y
  note: Z
  Vicon Raw : Inport
  Add1 : Sum  Inputs=-+
  Constant1 : Constant  Value=pi  OutDataTypeStr=double
  Demux : Demux  Outputs=6
  Flip_pi1 : Subsystem  mask(Flip -pi to pi){}
      mask help: Flips the inputs into the range -pi to pi
      mask Help: Flips the inputs into the range -pi to pi
      mask Display: disp('Flip_pi')
  Gain1 : Gain  Gain=0.001
  Gain3 : Gain  Gain=-1
  Gain6 : Gain  Gain=-0.001
  Gain7 : Gain  Gain=-0.001
  Matrix Concatenate1 : Concatenate  NumInputs=3  Mode=Multidimensional array
  Matrix Concatenate13 : Concatenate  NumInputs=3  Mode=Multidimensional array
  Position : Outport
  Attitude : Outport  Port=2
  wires:
  Constant1/1 -> Add1/2
  Demux/6 -> Matrix Concatenate1/3  "yaw"
  Gain1/1 -> Matrix Concatenate13/1
  Demux/1 -> Gain1/1
  Demux/2 -> Gain6/1
  Demux/3 -> Gain7/1
  Demux/4 -> Add1/1  "roll"
  Gain6/1 -> Matrix Concatenate13/2
  Gain7/1 -> Matrix Concatenate13/3
  Add1/1 -> Gain3/1
  Gain3/1 -> Flip_pi1/1(Angle)
  Demux/5 -> Matrix Concatenate1/2  "pitch"
  Flip_pi1/1(Angle_Flip) -> Matrix Concatenate1/1
  Matrix Concatenate13/1 -> Position/1
  Vicon Raw/1 -> Demux/1
  Matrix Concatenate1/1 -> Attitude/1

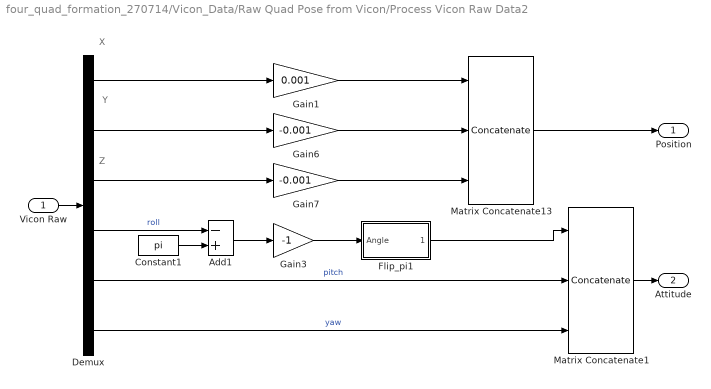
== system four_quad_formation_270714/Vicon_Data/Raw Quad Pose from Vicon/Process Vicon Raw Data2 ==
  note: Z
  note: Y
  note: X
  Vicon Raw : Inport
  Add1 : Sum  Inputs=-+
  Constant1 : Constant  Value=pi  OutDataTypeStr=double
  Demux : Demux  Outputs=6
  Flip_pi1 : Subsystem  mask(Flip -pi to pi){}
      mask help: Flips the inputs into the range -pi to pi
      mask Help: Flips the inputs into the range -pi to pi
      mask Display: disp('Flip_pi')
  Gain1 : Gain  Gain=0.001
  Gain3 : Gain  Gain=-1
  Gain6 : Gain  Gain=-0.001
  Gain7 : Gain  Gain=-0.001
  Matrix Concatenate1 : Concatenate  NumInputs=3  Mode=Multidimensional array
  Matrix Concatenate13 : Concatenate  NumInputs=3  Mode=Multidimensional array
  Position : Outport
  Attitude : Outport  Port=2
  wires:
  Matrix Concatenate1/1 -> Attitude/1
  Vicon Raw/1 -> Demux/1
  Matrix Concatenate13/1 -> Position/1
  Flip_pi1/1(Angle_Flip) -> Matrix Concatenate1/1
  Demux/5 -> Matrix Concatenate1/2  "pitch"
  Gain3/1 -> Flip_pi1/1(Angle)
  Add1/1 -> Gain3/1
  Gain7/1 -> Matrix Concatenate13/3
  Gain6/1 -> Matrix Concatenate13/2
  Demux/4 -> Add1/1  "roll"
  Demux/3 -> Gain7/1
  Demux/2 -> Gain6/1
  Demux/1 -> Gain1/1
  Gain1/1 -> Matrix Concatenate13/1
  Demux/6 -> Matrix Concatenate1/3  "yaw"
  Constant1/1 -> Add1/2

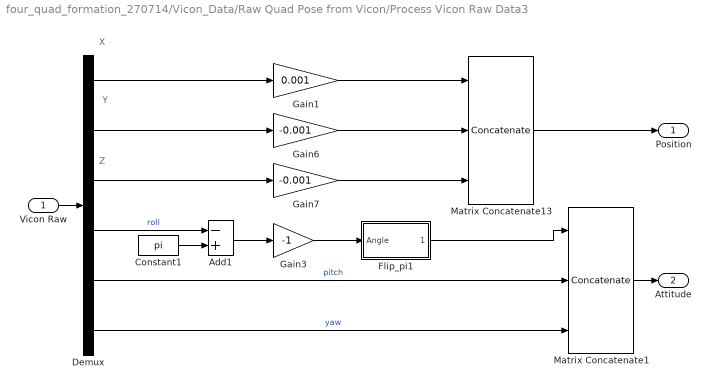
== system four_quad_formation_270714/Vicon_Data/Raw Quad Pose from Vicon/Process Vicon Raw Data3 ==
  note: Z
  note: Y
  note: X
  Vicon Raw : Inport
  Add1 : Sum  Inputs=-+
  Constant1 : Constant  Value=pi  OutDataTypeStr=double
  Demux : Demux  Outputs=6
  Flip_pi1 : Subsystem  mask(Flip -pi to pi){}
      mask help: Flips the inputs into the range -pi to pi
      mask Help: Flips the inputs into the range -pi to pi
      mask Display: disp('Flip_pi')
  Gain1 : Gain  Gain=0.001
  Gain3 : Gain  Gain=-1
  Gain6 : Gain  Gain=-0.001
  Gain7 : Gain  Gain=-0.001
  Matrix Concatenate1 : Concatenate  NumInputs=3  Mode=Multidimensional array
  Matrix Concatenate13 : Concatenate  NumInputs=3  Mode=Multidimensional array
  Position : Outport
  Attitude : Outport  Port=2
  wires:
  Matrix Concatenate1/1 -> Attitude/1
  Vicon Raw/1 -> Demux/1
  Matrix Concatenate13/1 -> Position/1
  Flip_pi1/1(Angle_Flip) -> Matrix Concatenate1/1
  Demux/5 -> Matrix Concatenate1/2  "pitch"
  Gain3/1 -> Flip_pi1/1(Angle)
  Add1/1 -> Gain3/1
  Gain7/1 -> Matrix Concatenate13/3
  Gain6/1 -> Matrix Concatenate13/2
  Demux/4 -> Add1/1  "roll"
  Demux/3 -> Gain7/1
  Demux/2 -> Gain6/1
  Demux/1 -> Gain1/1
  Gain1/1 -> Matrix Concatenate13/1
  Demux/6 -> Matrix Concatenate1/3  "yaw"
  Constant1/1 -> Add1/2

== system four_quad_formation_270714/Vicon_Data/Raw Quad Pose from Vicon/Process Vicon Raw Data4 ==
  note: X
  note: Y
  note: Z
  Vicon Raw : Inport
  Add1 : Sum  Inputs=-+
  Constant1 : Constant  Value=pi  OutDataTypeStr=double
  Demux : Demux  Outputs=6
  Flip_pi1 : Subsystem  mask(Flip -pi to pi){}
      mask help: Flips the inputs into the range -pi to pi
      mask Help: Flips the inputs into the range -pi to pi
      mask Display: disp('Flip_pi')
  Gain1 : Gain  Gain=0.001
  Gain3 : Gain  Gain=-1
  Gain6 : Gain  Gain=-0.001
  Gain7 : Gain  Gain=-0.001
  Matrix Concatenate1 : Concatenate  NumInputs=3  Mode=Multidimensional array
  Matrix Concatenate13 : Concatenate  NumInputs=3  Mode=Multidimensional array
  Position : Outport
  Attitude : Outport  Port=2
  wires:
  Constant1/1 -> Add1/2
  Demux/6 -> Matrix Concatenate1/3  "yaw"
  Gain1/1 -> Matrix Concatenate13/1
  Demux/1 -> Gain1/1
  Demux/2 -> Gain6/1
  Demux/3 -> Gain7/1
  Demux/4 -> Add1/1  "roll"
  Gain6/1 -> Matrix Concatenate13/2
  Gain7/1 -> Matrix Concatenate13/3
  Add1/1 -> Gain3/1
  Gain3/1 -> Flip_pi1/1(Angle)
  Demux/5 -> Matrix Concatenate1/2  "pitch"
  Flip_pi1/1(Angle_Flip) -> Matrix Concatenate1/1
  Matrix Concatenate13/1 -> Position/1
  Vicon Raw/1 -> Demux/1
  Matrix Concatenate1/1 -> Attitude/1

== system four_quad_formation_270714/Vicon_Data/Raw Quad Pose from Vicon/Process Vicon Raw Data1/Flip_pi1 ==
  Angle : Inport
  Add : Sum  Inputs=-+
  Compare To Constant1 : simulink/Logic and Bit Operations/Compare To Constant  relop=>  const=pi  OutDataTypeStr=uint8  ZeroCross=off
  Constant : Constant  Value=2*pi
  Data Type Duplicate : DataTypeDuplicate
  Flip_0_to_2pi : Subsystem  mask(Flip zero to 2pi){}
      mask help: Flips the inputs into the range zero to +2pi
      mask Help: Flips the inputs into the range zero to +2pi
      mask Display: disp('Flip_0_2pi')
  Switch : Switch  Criteria=u2 ~= 0
  Angle_Flip : Outport
  wires:
  Switch/1 -> Data Type Duplicate/1, Angle_Flip/1
  Add/1 -> Switch/1
  Constant/1 -> Add/1
  Compare To Constant1/1 -> Switch/2
  Flip_0_to_2pi/1(Angle_Flip) -> Add/2, Compare To Constant1/1, Switch/3
  Angle/1 -> Data Type Duplicate/2, Flip_0_to_2pi/1(Angle)

== system four_quad_formation_270714/Vicon_Data/Raw Quad Pose from Vicon/Process Vicon Raw Data2/Flip_pi1 ==
  Angle : Inport
  Add : Sum  Inputs=-+
  Compare To Constant1 : simulink/Logic and Bit Operations/Compare To Constant  relop=>  const=pi  OutDataTypeStr=uint8  ZeroCross=off
  Constant : Constant  Value=2*pi
  Data Type Duplicate : DataTypeDuplicate
  Flip_0_to_2pi : Subsystem  mask(Flip zero to 2pi){}
      mask help: Flips the inputs into the range zero to +2pi
      mask Help: Flips the inputs into the range zero to +2pi
      mask Display: disp('Flip_0_2pi')
  Switch : Switch  Criteria=u2 ~= 0
  Angle_Flip : Outport
  wires:
  Angle/1 -> Flip_0_to_2pi/1(Angle), Data Type Duplicate/2
  Flip_0_to_2pi/1(Angle_Flip) -> Switch/3, Compare To Constant1/1, Add/2
  Compare To Constant1/1 -> Switch/2
  Constant/1 -> Add/1
  Add/1 -> Switch/1
  Switch/1 -> Angle_Flip/1, Data Type Duplicate/1

== system four_quad_formation_270714/Vicon_Data/Raw Quad Pose from Vicon/Process Vicon Raw Data3/Flip_pi1 ==
  Angle : Inport
  Add : Sum  Inputs=-+
  Compare To Constant1 : simulink/Logic and Bit Operations/Compare To Constant  relop=>  const=pi  OutDataTypeStr=uint8  ZeroCross=off
  Constant : Constant  Value=2*pi
  Data Type Duplicate : DataTypeDuplicate
  Flip_0_to_2pi : Subsystem  mask(Flip zero to 2pi){}
      mask help: Flips the inputs into the range zero to +2pi
      mask Help: Flips the inputs into the range zero to +2pi
      mask Display: disp('Flip_0_2pi')
  Switch : Switch  Criteria=u2 ~= 0
  Angle_Flip : Outport
  wires:
  Angle/1 -> Flip_0_to_2pi/1(Angle), Data Type Duplicate/2
  Flip_0_to_2pi/1(Angle_Flip) -> Switch/3, Compare To Constant1/1, Add/2
  Compare To Constant1/1 -> Switch/2
  Constant/1 -> Add/1
  Add/1 -> Switch/1
  Switch/1 -> Angle_Flip/1, Data Type Duplicate/1

== system four_quad_formation_270714/Vicon_Data/Raw Quad Pose from Vicon/Process Vicon Raw Data4/Flip_pi1 ==
  Angle : Inport
  Add : Sum  Inputs=-+
  Compare To Constant1 : simulink/Logic and Bit Operations/Compare To Constant  relop=>  const=pi  OutDataTypeStr=uint8  ZeroCross=off
  Constant : Constant  Value=2*pi
  Data Type Duplicate : DataTypeDuplicate
  Flip_0_to_2pi : Subsystem  mask(Flip zero to 2pi){}
      mask help: Flips the inputs into the range zero to +2pi
      mask Help: Flips the inputs into the range zero to +2pi
      mask Display: disp('Flip_0_2pi')
  Switch : Switch  Criteria=u2 ~= 0
  Angle_Flip : Outport
  wires:
  Switch/1 -> Data Type Duplicate/1, Angle_Flip/1
  Add/1 -> Switch/1
  Constant/1 -> Add/1
  Compare To Constant1/1 -> Switch/2
  Flip_0_to_2pi/1(Angle_Flip) -> Add/2, Compare To Constant1/1, Switch/3
  Angle/1 -> Data Type Duplicate/2, Flip_0_to_2pi/1(Angle)

== system four_quad_formation_270714/Vicon_Data/Raw Quad Pose from Vicon/Process Vicon Raw Data1/Flip_pi1/Flip_0_to_2pi ==
  Angle : Inport
  Add : Sum
  Compare To Constant1 : simulink/Logic and Bit Operations/Compare To Constant  relop=<  const=0  OutDataTypeStr=uint8  ZeroCross=off
  Constant : Constant  Value=2*pi
  Data Type Duplicate : DataTypeDuplicate
  Flip_2pi : Subsystem  mask(Flip -2pi to 2pi){}
      mask help: Flips the inputs into the range -2pi to +2pi
      mask Help: Flips the inputs into the range -2pi to +2pi
      mask Display: disp('Flip_2pi')
  Switch : Switch  Criteria=u2 ~= 0
  Angle_Flip : Outport
  wires:
  Switch/1 -> Data Type Duplicate/1, Angle_Flip/1
  Angle/1 -> Data Type Duplicate/2, Flip_2pi/1(Angle)
  Add/1 -> Switch/1
  Constant/1 -> Add/1
  Compare To Constant1/1 -> Switch/2
  Flip_2pi/1(Angle_Flip) -> Switch/3, Add/2, Compare To Constant1/1

== system four_quad_formation_270714/Vicon_Data/Raw Quad Pose from Vicon/Process Vicon Raw Data2/Flip_pi1/Flip_0_to_2pi ==
  Angle : Inport
  Add : Sum
  Compare To Constant1 : simulink/Logic and Bit Operations/Compare To Constant  relop=<  const=0  OutDataTypeStr=uint8  ZeroCross=off
  Constant : Constant  Value=2*pi
  Data Type Duplicate : DataTypeDuplicate
  Flip_2pi : Subsystem  mask(Flip -2pi to 2pi){}
      mask help: Flips the inputs into the range -2pi to +2pi
      mask Help: Flips the inputs into the range -2pi to +2pi
      mask Display: disp('Flip_2pi')
  Switch : Switch  Criteria=u2 ~= 0
  Angle_Flip : Outport
  wires:
  Flip_2pi/1(Angle_Flip) -> Compare To Constant1/1, Add/2, Switch/3
  Compare To Constant1/1 -> Switch/2
  Constant/1 -> Add/1
  Add/1 -> Switch/1
  Angle/1 -> Flip_2pi/1(Angle), Data Type Duplicate/2
  Switch/1 -> Angle_Flip/1, Data Type Duplicate/1

== system four_quad_formation_270714/Vicon_Data/Raw Quad Pose from Vicon/Process Vicon Raw Data3/Flip_pi1/Flip_0_to_2pi ==
  Angle : Inport
  Add : Sum
  Compare To Constant1 : simulink/Logic and Bit Operations/Compare To Constant  relop=<  const=0  OutDataTypeStr=uint8  ZeroCross=off
  Constant : Constant  Value=2*pi
  Data Type Duplicate : DataTypeDuplicate
  Flip_2pi : Subsystem  mask(Flip -2pi to 2pi){}
      mask help: Flips the inputs into the range -2pi to +2pi
      mask Help: Flips the inputs into the range -2pi to +2pi
      mask Display: disp('Flip_2pi')
  Switch : Switch  Criteria=u2 ~= 0
  Angle_Flip : Outport
  wires:
  Flip_2pi/1(Angle_Flip) -> Compare To Constant1/1, Add/2, Switch/3
  Compare To Constant1/1 -> Switch/2
  Constant/1 -> Add/1
  Add/1 -> Switch/1
  Angle/1 -> Flip_2pi/1(Angle), Data Type Duplicate/2
  Switch/1 -> Angle_Flip/1, Data Type Duplicate/1

== system four_quad_formation_270714/Vicon_Data/Raw Quad Pose from Vicon/Process Vicon Raw Data4/Flip_pi1/Flip_0_to_2pi ==
  Angle : Inport
  Add : Sum
  Compare To Constant1 : simulink/Logic and Bit Operations/Compare To Constant  relop=<  const=0  OutDataTypeStr=uint8  ZeroCross=off
  Constant : Constant  Value=2*pi
  Data Type Duplicate : DataTypeDuplicate
  Flip_2pi : Subsystem  mask(Flip -2pi to 2pi){}
      mask help: Flips the inputs into the range -2pi to +2pi
      mask Help: Flips the inputs into the range -2pi to +2pi
      mask Display: disp('Flip_2pi')
  Switch : Switch  Criteria=u2 ~= 0
  Angle_Flip : Outport
  wires:
  Switch/1 -> Data Type Duplicate/1, Angle_Flip/1
  Angle/1 -> Data Type Duplicate/2, Flip_2pi/1(Angle)
  Add/1 -> Switch/1
  Constant/1 -> Add/1
  Compare To Constant1/1 -> Switch/2
  Flip_2pi/1(Angle_Flip) -> Switch/3, Add/2, Compare To Constant1/1

== system four_quad_formation_270714/Vicon_Data/Raw Quad Pose from Vicon/Process Vicon Raw Data1/Flip_pi1/Flip_0_to_2pi/Flip_2pi ==
  Angle : Inport
  Bias : Bias  Bias=-2*pi
  Constant : Constant  Value=2*pi
  Data Type Duplicate : DataTypeDuplicate
  Modulo : Math  Operator=mod  SaturateOnIntegerOverflow=on
  Sign1 : Signum
  Switch : Switch
  Angle_Flip : Outport
  wires:
  Switch/1 -> Data Type Duplicate/2, Angle_Flip/1
  Bias/1 -> Switch/3
  Sign1/1 -> Switch/2
  Modulo/1 -> Switch/1, Bias/1
  Constant/1 -> Modulo/2
  Angle/1 -> Data Type Duplicate/1, Sign1/1, Modulo/1

== system four_quad_formation_270714/Vicon_Data/Raw Quad Pose from Vicon/Process Vicon Raw Data2/Flip_pi1/Flip_0_to_2pi/Flip_2pi ==
  Angle : Inport
  Bias : Bias  Bias=-2*pi
  Constant : Constant  Value=2*pi
  Data Type Duplicate : DataTypeDuplicate
  Modulo : Math  Operator=mod  SaturateOnIntegerOverflow=on
  Sign1 : Signum
  Switch : Switch
  Angle_Flip : Outport
  wires:
  Angle/1 -> Modulo/1, Sign1/1, Data Type Duplicate/1
  Constant/1 -> Modulo/2
  Modulo/1 -> Bias/1, Switch/1
  Sign1/1 -> Switch/2
  Bias/1 -> Switch/3
  Switch/1 -> Angle_Flip/1, Data Type Duplicate/2

== system four_quad_formation_270714/Vicon_Data/Raw Quad Pose from Vicon/Process Vicon Raw Data3/Flip_pi1/Flip_0_to_2pi/Flip_2pi ==
  Angle : Inport
  Bias : Bias  Bias=-2*pi
  Constant : Constant  Value=2*pi
  Data Type Duplicate : DataTypeDuplicate
  Modulo : Math  Operator=mod  SaturateOnIntegerOverflow=on
  Sign1 : Signum
  Switch : Switch
  Angle_Flip : Outport
  wires:
  Angle/1 -> Modulo/1, Sign1/1, Data Type Duplicate/1
  Constant/1 -> Modulo/2
  Modulo/1 -> Bias/1, Switch/1
  Sign1/1 -> Switch/2
  Bias/1 -> Switch/3
  Switch/1 -> Angle_Flip/1, Data Type Duplicate/2

== system four_quad_formation_270714/Vicon_Data/Raw Quad Pose from Vicon/Process Vicon Raw Data4/Flip_pi1/Flip_0_to_2pi/Flip_2pi ==
  Angle : Inport
  Bias : Bias  Bias=-2*pi
  Constant : Constant  Value=2*pi
  Data Type Duplicate : DataTypeDuplicate
  Modulo : Math  Operator=mod  SaturateOnIntegerOverflow=on
  Sign1 : Signum
  Switch : Switch
  Angle_Flip : Outport
  wires:
  Switch/1 -> Data Type Duplicate/2, Angle_Flip/1
  Bias/1 -> Switch/3
  Sign1/1 -> Switch/2
  Modulo/1 -> Switch/1, Bias/1
  Constant/1 -> Modulo/2
  Angle/1 -> Data Type Duplicate/1, Sign1/1, Modulo/1

== stateflow chart four_quad_formation_270714/Subsystem/Trajectory Logic/ SF ==
  state Airborne
    state Stage6
      state Red_UAV1 [parallel]
        du:PosDes_UAV1[0] = -1.457;
        PosDes_UAV1[1] = 1.457 ;
        PosDes_UAV1[2] = -1.2;
        settings: executionOrder=1
      state Green_UAV2 [parallel]
        du:PosDes_UAV2[0] = 1.457 ;
        PosDes_UAV2[1] = 1.457;
        PosDes_UAV2[2] = -1.2;
        settings: executionOrder=2
      state PWM1 [parallel]
        du:    Increm = Increm + DeltaT
        settings: executionOrder=3
      state PWM [parallel]
        du:    pwm=  1800;
        settings: executionOrder=4
      state Blue_UAV3 [parallel]
        du:PosDes_UAV3[0] = -1.457  ;
        PosDes_UAV3[1] = -1.457;
        PosDes_UAV3[2] = -1.2;
        settings: executionOrder=5
      state Purple_UAV4 [parallel]
        du:PosDes_UAV4[0] = 1.457 ;
        PosDes_UAV4[1] = -1.457;
        PosDes_UAV4[2] = -1.2;
        settings: executionOrder=6
    state TakeOff
      du:		HoverThrottle = (H0 - HoverThrottle)*2*DeltaT + HoverThrottle ;
      PosDes_UAV1[2] = (-1.2 - PosDes_UAV1[2])*1*DeltaT + PosDes_UAV1[2] ;
      PosDes_UAV2[2] = (-1.2 - PosDes_UAV2[2])*1*DeltaT + PosDes_UAV2[2] ;
      PosDes_UAV3[2] = (-1.2 - PosDes_UAV3[2])*1*DeltaT + PosDes_UAV3[2] ;
      PosDes_UAV4[2] = (-1.2 - PosDes_UAV4[2])*1*DeltaT + PosDes_UAV4[2] ;
    state Stage1
      state Red_UAV1 [parallel]
        du:PosDes_UAV1[0] = (2- PosDes_UAV1[0])*0.75*DeltaT + PosDes_UAV1[0] ;
        PosDes_UAV1[1] = (2- PosDes_UAV1[1])*0.75*DeltaT + PosDes_UAV1[1] ;
        PosDes_UAV1[2] = (-1.2- PosDes_UAV1[2])*0.75*DeltaT + PosDes_UAV1[2] ;
        settings: executionOrder=1
      state Green_UAV2 [parallel]
        du:PosDes_UAV2[0] = (-2-PosDes_UAV2[0])*0.75*DeltaT+PosDes_UAV2[0];
        PosDes_UAV2[1] = (2-PosDes_UAV2[1])*0.75*DeltaT+PosDes_UAV2[1];
        PosDes_UAV2[2] = (-1.2-PosDes_UAV2[2])*0.75*DeltaT+PosDes_UAV2[2];
        settings: executionOrder=2
      state PWM [parallel]
        du:    pwm=  1800;
        settings: executionOrder=3
      state Blue_UAV3 [parallel]
        du:PosDes_UAV3[0] = (2-PosDes_UAV3[0])*0.75*DeltaT + PosDes_UAV3[0];
        PosDes_UAV3[1] = (-2-PosDes_UAV3[1])*0.75*DeltaT+PosDes_UAV3[1];
        PosDes_UAV3[2] = (-1.2-PosDes_UAV3[2])*0.75*DeltaT+PosDes_UAV3[2];
        settings: executionOrder=4
      state Purple_UAV4 [parallel]
        du:PosDes_UAV4[0] = (-2-PosDes_UAV4[0])*0.75*DeltaT + PosDes_UAV4[0];
        PosDes_UAV4[1] = (-2-PosDes_UAV4[1])*0.75*DeltaT+PosDes_UAV4[1];
        PosDes_UAV4[2] = (-1.2-PosDes_UAV4[2])*0.75*DeltaT+PosDes_UAV4[2];
        settings: executionOrder=5
    state Stage7
      state Red_UAV1 [parallel]
        du:PosDes_UAV1[0] = 3.5*cos(81.087*PI/180-Increm*omega_circle)-2;
        PosDes_UAV1[1] = 3.5*sin(81.087*PI/180-Increm*omega_circle)-2 ;
        PosDes_UAV1[2] = -1.2;
        settings: executionOrder=1
      state Green_UAV2 [parallel]
        du:PosDes_UAV2[0] = 3.5*cos(351.087*PI/180-Increm*omega_circle)-2;
        PosDes_UAV2[1] = 3.5*sin(351.087*PI/180-Increm*omega_circle)+2;
        PosDes_UAV2[2] = -1.2;
        settings: executionOrder=2
      state PWM1 [parallel]
        du:    Increm = Increm + DeltaT
        settings: executionOrder=3
      state PWM [parallel]
        du:    pwm=  1800;
        settings: executionOrder=4
      state Blue_UAV3 [parallel]
        du:PosDes_UAV3[0] = 3.5*cos(171.087*PI/180-Increm*omega_circle)+2  ;
        PosDes_UAV3[1] = 3.5*sin(171.087*PI/180-Increm*omega_circle)-2;
        PosDes_UAV3[2] = -1.2;
        settings: executionOrder=5
      state Purple_UAV4 [parallel]
        du:PosDes_UAV4[0] = 3.5*cos(261.087*PI/180-Increm*omega_circle)+2 ;
        PosDes_UAV4[1] = 3.5*sin(261.087*PI/180-Increm*omega_circle)+2;
        PosDes_UAV4[2] = -1.2;
        settings: executionOrder=6
    state Stage2
      state Red_UAV1 [parallel]
        du:PosDes_UAV1[0] = 2-Increm ;
        PosDes_UAV1[1] = 2 ;
        PosDes_UAV1[2] = -1.2 ;
        settings: executionOrder=1
      state Green_UAV2 [parallel]
        du:PosDes_UAV2[0] = -2+Increm;
        PosDes_UAV2[1] = 2;
        PosDes_UAV2[2] = -1.2;
        settings: executionOrder=2
      state PWM2 [parallel]
        du:    Increm = Increm + DeltaT
        settings: executionOrder=3
      state PWM [parallel]
        du:    pwm=  1800;
        settings: executionOrder=4
      state Blue_UAV3 [parallel]
        du:PosDes_UAV3[0] = 2- Increm;
        PosDes_UAV3[1] = -2;
        PosDes_UAV3[2] = -1.2;
        settings: executionOrder=5
      state Purple_UAV4 [parallel]
        du:PosDes_UAV4[0] = -2+Increm;
        PosDes_UAV4[1] = -2;
        PosDes_UAV4[2] = -1.2;
        settings: executionOrder=6
    state Stage8
      state Red_UAV1 [parallel]
        du:PosDes_UAV1[0] = 2;
        PosDes_UAV1[1] = -2;
        PosDes_UAV1[2] = -1.2;
        settings: executionOrder=1
      state Green_UAV2 [parallel]
        du:PosDes_UAV2[0] = -2;
        PosDes_UAV2[1] = -2;
        PosDes_UAV2[2] = -1.2;
        settings: executionOrder=2
      state PWM1 [parallel]
        du:    Increm = Increm + DeltaT
        settings: executionOrder=3
      state PWM [parallel]
        du:    pwm=  1800;
        settings: executionOrder=4
      state Blue_UAV3 [parallel]
        du:PosDes_UAV3[0] = 2 ;
        PosDes_UAV3[1] = 2;
        PosDes_UAV3[2] = -1.2;
        settings: executionOrder=5
      state Purple_UAV4 [parallel]
        du:PosDes_UAV4[0] = -2;
        PosDes_UAV4[1] = 2;
        PosDes_UAV4[2] = -1.2;
        settings: executionOrder=6
    state Stage3
      state Red_UAV1 [parallel]
        du:PosDes_UAV1[0] = 0.8-Increm ;
        PosDes_UAV1[1] = 0.625*(0.8-Increm)*(0.8-Increm)+1.6 ;
        PosDes_UAV1[2] = -1.2;
        settings: executionOrder=1
      state Green_UAV2 [parallel]
        du:PosDes_UAV2[0] = -0.8+Increm;
        PosDes_UAV2[1] = -0.625*(0.8-Increm)*(0.8-Increm)+2.4;
        PosDes_UAV2[2] = -1.2;
        settings: executionOrder=2
      state PWM1 [parallel]
        du:    Increm = Increm + DeltaT
        settings: executionOrder=3
      state PWM [parallel]
        du:    pwm=  1800;
        settings: executionOrder=4
      state Blue_UAV3 [parallel]
        du:PosDes_UAV3[0] = 0.8-Increm;
        PosDes_UAV3[1] = 0.625*(0.8-Increm)*(0.8-Increm)-2.4;
        PosDes_UAV3[2] = -1.2;
        settings: executionOrder=5
      state Purple_UAV4 [parallel]
        du:PosDes_UAV4[0] = -0.8+Increm;
        PosDes_UAV4[1] = -0.625*(0.8-Increm)*(0.8-Increm)-1.6;
        PosDes_UAV4[2] = -1.2;
        settings: executionOrder=6
    state Stage9
      state Red_UAV1 [parallel]
        du:PosDes_UAV1[0] = 0;
        PosDes_UAV1[1] = -2;
        PosDes_UAV1[2] = -1.2;
        settings: executionOrder=1
      state Green_UAV2 [parallel]
        du:PosDes_UAV2[0] = 0;
        PosDes_UAV2[1] = -0.75;
        PosDes_UAV2[2] = -1.2;
        settings: executionOrder=2
      state PWM1 [parallel]
        du:    Increm = Increm + DeltaT
        settings: executionOrder=3
      state PWM [parallel]
        du:    pwm=  1800;
        settings: executionOrder=4
      state Blue_UAV3 [parallel]
        du:PosDes_UAV3[0] = 0 ;
        PosDes_UAV3[1] = 0.75;
        PosDes_UAV3[2] = -1.2;
        settings: executionOrder=5
      state Purple_UAV4 [parallel]
        du:PosDes_UAV4[0] = 0;
        PosDes_UAV4[1] = 2;
        PosDes_UAV4[2] = -1.2;
        settings: executionOrder=6
    state Stage4
      state Red_UAV1 [parallel]
        du:PosDes_UAV1[0] = -0.8-Increm;
        PosDes_UAV1[1] = 2 ;
        PosDes_UAV1[2] = -1.2;
        settings: executionOrder=1
      state Green_UAV2 [parallel]
        du:PosDes_UAV2[0] = 0.8+ Increm ;
        PosDes_UAV2[1] = 2;
        PosDes_UAV2[2] = -1.2;
        settings: executionOrder=2
      state PWM1 [parallel]
        du:    Increm = Increm + DeltaT
        settings: executionOrder=3
      state PWM [parallel]
        du:    pwm=  1800;
        settings: executionOrder=4
      state Blue_UAV3 [parallel]
        du:PosDes_UAV3[0] = -0.8- Increm  ;
        PosDes_UAV3[1] = -2;
        PosDes_UAV3[2] = -1.2;
        settings: executionOrder=5
      state Purple_UAV4 [parallel]
        du:PosDes_UAV4[0] = 0.8 + Increm ;
        PosDes_UAV4[1] = -2;
        PosDes_UAV4[2] = -1.2;
        settings: executionOrder=6
    state Stage10
      state Red_UAV1 [parallel]
        du:PosDes_UAV1[0] = 2*cos(180*PI/180-Increm*omega_circle);
        PosDes_UAV1[1] =  2*sin(180*PI/180-Increm*omega_circle);
        PosDes_UAV1[2] = -1.2;
        settings: executionOrder=1
      state Green_UAV2 [parallel]
        du:PosDes_UAV2[0] = 0.75*cos(180*PI/180-Increm*omega_circle);
        PosDes_UAV2[1] = 0.75*sin(180*PI/180-Increm*omega_circle);
        PosDes_UAV2[2] = -1.2;
        settings: executionOrder=2
      state PWM1 [parallel]
        du:    Increm = Increm + DeltaT
        settings: executionOrder=3
      state PWM [parallel]
        du:    pwm=  1800;
        settings: executionOrder=4
      state Blue_UAV3 [parallel]
        du:PosDes_UAV3[0] = 0.75*cos(0*PI/180-Increm*omega_circle) ;
        PosDes_UAV3[1] = 0.75*sin(0*PI/180-Increm*omega_circle);
        PosDes_UAV3[2] = -1.2;
        settings: executionOrder=5
      state Purple_UAV4 [parallel]
        du:PosDes_UAV4[0] = 2*cos(0*PI/180-Increm*omega_circle);
        PosDes_UAV4[1] = 2*sin(0*PI/180-Increm*omega_circle);
        PosDes_UAV4[2] = -1.2;
        settings: executionOrder=6
    state Stage5
      state Red_UAV1 [parallel]
        du:PosDes_UAV1[0] = -2;
        PosDes_UAV1[1] = 2 ;
        PosDes_UAV1[2] = -1.2;
        settings: executionOrder=1
      state Green_UAV2 [parallel]
        du:PosDes_UAV2[0] = 2 ;
        PosDes_UAV2[1] = 2;
        PosDes_UAV2[2] = -1.2;
        settings: executionOrder=2
      state PWM1 [parallel]
        du:    Increm = Increm + DeltaT
        settings: executionOrder=3
      state PWM [parallel]
        du:    pwm=  1800;
        settings: executionOrder=4
      state Blue_UAV3 [parallel]
        du:PosDes_UAV3[0] = -2  ;
        PosDes_UAV3[1] = -2;
        PosDes_UAV3[2] = -1.2;
        settings: executionOrder=5
      state Purple_UAV4 [parallel]
        du:PosDes_UAV4[0] = 2 ;
        PosDes_UAV4[1] = -2;
        PosDes_UAV4[2] = -1.2;
        settings: executionOrder=6
    state Stage11
      state Red_UAV1 [parallel]
        du:PosDes_UAV1[0] = 2;
        PosDes_UAV1[1] = 0;
        PosDes_UAV1[2] = -1.2;
        settings: executionOrder=1
      state Green_UAV2 [parallel]
        du:PosDes_UAV2[0] = 0.75;
        PosDes_UAV2[1] = 0;
        PosDes_UAV2[2] = -1.2;
        settings: executionOrder=2
      state PWM1 [parallel]
        du:    Increm = Increm + DeltaT
        settings: executionOrder=3
      state PWM [parallel]
        du:    pwm=  1800;
        settings: executionOrder=4
      state Blue_UAV3 [parallel]
        du:PosDes_UAV3[0] = -0.75 ;
        PosDes_UAV3[1] = 0;
        PosDes_UAV3[2] = -1.2;
        settings: executionOrder=5
      state Purple_UAV4 [parallel]
        du:PosDes_UAV4[0] = -2;
        PosDes_UAV4[1] = 0;
        PosDes_UAV4[2] = -1.2;
        settings: executionOrder=6
    (default) -> TakeOff : {	PosDes_UAV1 = Pos_UAV1;
        | 	PosDes_UAV2 = Pos_UAV2;
        | 	PosDes_UAV3 = Pos_UAV3;
        | 	PosDes_UAV4 = Pos_UAV4;
        | 	 }
    Stage5 -> Stage6 : after(3,sec)
    TakeOff -> Stage1 : after (3, sec)
    Stage6 -> Stage7 : [(abs(Pos_UAV1[0]-(-1.457)))<0.1]
        | {Increm = 0;}
    Stage1 -> Stage2 : after (3, sec)
        | {Increm =0;}
    Stage7 -> Stage8 : [(abs(Pos_UAV1[0]-1.457))<0.2]
        | {Increm = 0;}
    Stage2 -> Stage3 : [(abs(Pos_UAV1[0]-0.8))<0.1]
        | {Increm = 0;}
    Stage8 -> Stage9 : after (3,sec)
        | {Increm = 0;}
    Stage3 -> Stage4 : [(abs(Pos_UAV1[0]-(-0.8)))<0.1]
        | {Increm = 0;}
    Stage9 -> Stage10 : after (5, sec)
        | {Increm =0;}
    Stage4 -> Stage5 : [(abs(Pos_UAV1[0]-(-2)))<0.1]
        | {Increm = 0;}
    Stage10 -> Stage11 : [(abs(Pos_UAV1[0]-2))<0.1]
  state Landing
    state Decsending
      en:		PosDes_UAV1 = Pos_UAV1;	PosDes_UAV2 = Pos_UAV2;  PosDes_UAV3 = Pos_UAV3;
      PosDes_UAV4 = Pos_UAV4;
      du:		PosDes_UAV1[2] = (0 - PosDes_UAV1[2])*0.2*DeltaT + PosDes_UAV1[2] ;
      PosDes_UAV2[2] = (0 - PosDes_UAV2[2])*0.2*DeltaT + PosDes_UAV2[2] ;
      PosDes_UAV3[2] = (0 - PosDes_UAV3[2])*0.2*DeltaT + PosDes_UAV3[2] ;
      PosDes_UAV4[2] = (0 - PosDes_UAV4[2])*0.2*DeltaT + PosDes_UAV4[2] ;
    state CutThrottle
      du:		HoverThrottle = (0.0 - HoverThrottle)*3*DeltaT + HoverThrottle ;
    (default) -> Decsending
    Decsending -> (junction 288) : after(2,sec)
    (junction 288) -> CutThrottle : [Pos_UAV1[2] > -0.2]
  Landing -> Airborne : [RC[6] > 0.5]
  Airborne -> Landing : [RC[6] < -0.5]
  (default) -> Landing : {HoverThrottle=0.0}
  data: HoverThrottle output double size=1; PosDes_UAV1 output double size=4; PosDes_UAV2 output double size=4; PosDes_UAV3 output double size=4; RC input size=8; Pos_UAV1 input size=4; DeltaT parameter size=1; H0 parameter size=1; Kl parameter size=1; Increm local double size=1; omega_circle parameter size=1; PI parameter size=1; omega_h parameter; Circle_R parameter size=1; MAX_Height parameter size=1; Pos_UAV2 input size=4; Pos_UAV3 input size=4; Pos_UAV4 input size=4; PosDes_UAV4 output double size=4; pwm output double
